simulink model "feeder_1_3_ss_pmu"  (Simulink 9.2)
settings: Solver=ode4  StartTime=0.0  StopTime=inf  FixedStep=0.0001  RelTol=1e-3
PreLoadFcn:
  | Ts=100e-6;Core_Num = 0;
PostLoadFcn:
  | Ts=100e-6;Core_Num = 0;
InitFcn:
  | Ts=100e-6;Core_Num = 0;
libraries: powerlib_meascontrol x153, rtio_generic_c37_118 x17, simulink x17, artemis x2, opal_lib x2, rtlab x1, powerlib x1
(part 4 of 4)

== system feeder_1_3_ss_pmu/SS_PMU/Subsystem9/Subsystem/Subsystem1/Subsystem ==
  Measurements1 : Inport
  Constant : Constant  Value=3
  Demux1 : Demux  Outputs=6
  Discrete Derivative : simulink/Discrete/Discrete Derivative  gainval=1.0  ICPrevScaledInput=0.0  OutMin=[]  OutMax=[]  OutDataType=fixdt(1, 16)  OutScaling=2^-10  DoSatur=off
  Display : Display
  Display1 : Display
  Divide : Product  Inputs=*/
  Fourier{1..6} (6 alike) : powerlib_meascontrol/Measurements/Fourier  Freq=60  n=1  InInit=[0, 0]  Ts=Ts
      settings: SourceProductName=Simscape Power Systems
  Gain{,1..5} (6 alike) : Gain  Gain=1/sqrt(2)
  Mux : Mux  Inputs=6
  Mux{2..4,6..8} (6 alike) : Mux  Inputs=2
  Mux5 : Mux  Inputs=3
  PLL : powerlib_meascontrol/PLL/PLL  Fmin=60  Par_Init=[0, 60]  ParK=[180, 3200, 1]  TcD=1.6e-4  MaxRateChangeFreq=12  FilterCutOffFreq=25  Ts=Ts  AGC=on
      settings: SourceProductName=Simscape Power Systems  SourceProductBaseCode=PS
  PLL1 : powerlib_meascontrol/PLL/PLL  Fmin=60  Par_Init=[0, 60]  ParK=[180, 3200, 1]  TcD=1.6e-4  MaxRateChangeFreq=12  FilterCutOffFreq=25  Ts=Ts  AGC=on
      settings: SourceProductName=Simscape Power Systems  SourceProductBaseCode=PS
  PLL2 : powerlib_meascontrol/PLL/PLL  Fmin=60  Par_Init=[0, 60]  ParK=[180, 3200, 1]  TcD=1.6e-4  MaxRateChangeFreq=12  FilterCutOffFreq=25  Ts=Ts  AGC=on
      settings: SourceProductName=Simscape Power Systems  SourceProductBaseCode=PS
  Sum of Elements : Sum  Inputs=+
  Terminator : Terminator
  Terminator1 : Terminator
  Terminator2 : Terminator
  Phasors_60Hz : Outport
  Phasors_freq : Outport  Port=2
  Phasors_dtfreq1 : Outport  Port=3
  wires:
  Mux5/1 -> Sum of Elements/1
  PLL2/1 -> Mux5/3
  PLL1/1 -> Mux5/2
  PLL/1 -> Mux5/1
  PLL2/2 -> Terminator2/1
  PLL1/2 -> Terminator1/1
  PLL/2 -> Terminator/1
  [Vc] -> PLL2/1
  [Vb] -> PLL1/1
  [Va] -> PLL/1
  Discrete Derivative/1 -> Display1/1, Phasors_dtfreq1/1
  Mux3/1 -> Mux/2
  Mux2/1 -> Mux/1
  Demux1/2 -> [Vb]
  Measurements1/1 -> Demux1/1
  [Va] -> Fourier2/1
  Demux1/3 -> [Vc]
  Demux1/1 -> [Va]
  Mux7/1 -> Mux/5
  Mux4/1 -> Mux/3
  Mux/1 -> Phasors_60Hz/1
  Demux1/4 -> [Ia]
  Demux1/6 -> [Ic]
  Demux1/5 -> [Ib]
  Mux8/1 -> Mux/6
  Mux6/1 -> Mux/4
  Sum of Elements/1 -> Divide/1
  Divide/1 -> Display/1, Discrete Derivative/1, Phasors_freq/1
  Constant/1 -> Divide/2
  Fourier2/2 -> Mux2/2
  [Vc] -> Fourier3/1
  [Ia] -> Fourier4/1
  Fourier2/1 -> Gain/1
  Gain/1 -> Mux2/1
  [Vb] -> Fourier1/1
  Fourier1/2 -> Mux3/2
  Fourier1/1 -> Gain1/1
  Gain1/1 -> Mux3/1
  Fourier3/2 -> Mux4/2
  Fourier3/1 -> Gain2/1
  Gain2/1 -> Mux4/1
  Fourier4/2 -> Mux6/2
  Fourier4/1 -> Gain3/1
  Gain3/1 -> Mux6/1
  Fourier5/2 -> Mux7/2
  Fourier5/1 -> Gain4/1
  Gain4/1 -> Mux7/1
  Fourier6/2 -> Mux8/2
  Fourier6/1 -> Gain5/1
  Gain5/1 -> Mux8/1
  [Ic] -> Fourier6/1
  [Ib] -> Fourier5/1
